simulink model "consignas"  (R2018a)
settings: Solver=VariableStepAuto  StartTime=0.0  StopTime=30  RelTol=1e-3
libraries: simulink x4
settings Model: Creator=wafle  LastModifiedBy=wafle

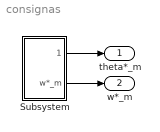
== system consignas ==
  Subsystem : Subsystem
  theta*_m : Outport
  w*_m : Outport  Port=2
  wires:
  Subsystem/1(theta*_m) -> theta*_m/1
  Subsystem/2(w*_m) -> w*_m/1

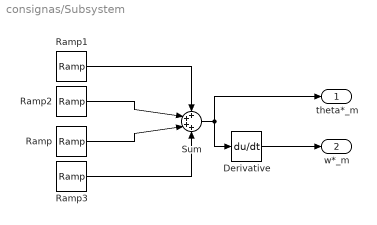
== system consignas/Subsystem ==
  Derivative : Derivative
  Ramp : simulink/Sources/Ramp  slope=-2*pi/5  start=15  InitialOutput=0
  Ramp1 : simulink/Sources/Ramp  slope=2*pi/5  start=5  InitialOutput=0
  Ramp2 : simulink/Sources/Ramp  slope=-2*pi/5  start=10  InitialOutput=0
  Ramp3 : simulink/Sources/Ramp  slope=2*pi/5  start=20  InitialOutput=0
  Sum : Sum  Inputs=4
  theta*_m : Outport
  w*_m : Outport  Port=2
  wires:
  Ramp1/1 -> Sum/1
  Sum/1 -> theta*_m/1, Derivative/1
  Ramp2/1 -> Sum/2
  Derivative/1 -> w*_m/1
  Ramp/1 -> Sum/3
  Ramp3/1 -> Sum/4
